simulink model "untitled"  (R2021a)
settings: Solver=VariableStepAuto  StartTime=0.0  StopTime=10.0  RelTol=1e-3
settings Model: Creator=Gooooood  LastModifiedBy=Gooooood

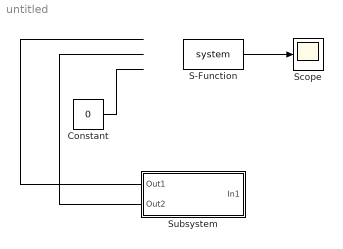
== system untitled ==
  Constant : Constant  Value=0
  S-Function : S-Function  SFunctionDeploymentMode=off  EnableBusSupport=off
  Scope : Scope
  Subsystem : Subsystem
  wires:
  Constant/1 -> ?
  Subsystem/2(Out2) -> ?
  Subsystem/1(Out1) -> ?
  S-Function/1 -> Scope/1

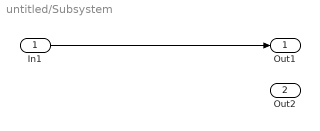
== system untitled/Subsystem ==
  In1 : Inport
  Out1 : Outport
  Out2 : Outport  Port=2
  wires:
  In1/1 -> Out1/1
